simulink model "tutorial_vms"  (R2023a)
settings: Solver=FixedStepAuto  StartTime=0.0  StopTime=50  FixedStep=framePeriod_s  RelTol=1e-3
undefined symbols (not defined in the file): Aircraft, framePeriod_s
settings Model: Creator=brian  LastModifiedBy=tuan
settings SolverCC: AlgebraicLoopSolver=TrustRegion
settings OptimizationCC: DefaultParameterBehavior=Inlined  GainParamInheritBuiltInType=on  UseFloatMulNetSlope=on  DefaultUnderspecifiedDataType=single  EnhancedBackFolding=on  BooleansAsBitfields=on  PassReuseOutputArgsAs=Individual arguments  StateBitsets=on  DataBitsets=on  ActiveStateOutputEnumStorageType=uint16  ZeroExternalMemoryAtStartup=off  ZeroInternalMemoryAtStartup=off  EfficientFloat2IntCast=on  LifeSpan=inf  DifferentSizesBufferReuse=on  OptimizationPriority=RAM  OptimizationCustomize=off  EfficientTunableParamExpr=on
settings DebuggingCC: ParameterPrecisionLossMsg=none  ParameterTunabilityLossMsg=error  UnconnectedInputMsg=warning  UnconnectedOutputMsg=warning  UnconnectedLineMsg=warning  BusObjectLabelMismatch=error  RootOutportRequireBusObject=error  NonBusSignalsTreatedAsBus=error  SFInvalidInputDataAccessInChartInitDiag=error  SFTransitionOutsideNaturalParentDiag=error  SFUnreachableExecutionPathDiag=error  SFUndirectedBroadcastEventsDiag=error
settings HardwareCC: ProdBitPerPointer=32  ProdBitPerSizeT=32  ProdBitPerPtrDiffT=32  ProdLargestAtomicInteger=Long  ProdLargestAtomicFloat=Double  ProdWordSize=32  ProdHWDeviceType=NXP->Cortex-M4  TargetLargestAtomicInteger=Long  TargetLargestAtomicFloat=Double  TargetLongLongMode=on  TargetIntDivRoundTo=Zero  TargetEndianess=LittleEndian  TargetHWDeviceType=NXP->Cortex-M4  ProdEqTarget=off
settings ModelReferenceCC: EnableRefExpFcnMdlSchedulingChecks=on  ModelReferenceNumInstancesAllowed=Single
settings SFSimCC: SimParseCustomCode=off  SimGenImportedTypeDefs=on  MATLABDynamicMemAlloc=off  SimTargetLang=C++
settings SFSimCC: SimUserIncludeDirs=|
  | ../../flight_code/include
  | ../../../ua_spaaro_extra/imu/include
  | ../../../ua_spaaro_extra/gnss/include
  | ../../../ua_spaaro_extra/pres/include
  | ../../../ua_spaaro_extra/sbus/include
  | ../../../ua_spaaro_extra/global_defs/include
settings SFSimCC: SimUserDefines=|
  | SIL
  | __FMU_R_MINI_V1__
settings RTWCC: Description=Embedded Coder  SystemTargetFile=ert.tlc  GenCodeOnly=on  TemplateMakefile=ert_default_tmf  GenerateReport=on  RTWVerbose=off  RTWUseSimCustomCode=on  Toolchain=GNU gcc/g++ | gmake (64-bit Linux)  BuildConfiguration=Specify  IncludeHyperlinkInReport=on  LaunchReport=on  TargetLang=C++  GenerateTraceInfo=on  GenerateTraceReport=on  GenerateTraceReportSl=on  GenerateTraceReportSf=on  GenerateTraceReportEml=on  GenerateCodeReplacementReport=on  DLArmComputeVersion=19.05
settings RTWCC: CustomInclude=|
  | ../../flight_code/include
  | ../../../ua_spaaro_extra/imu/include
  | ../../../ua_spaaro_extra/gnss/include
  | ../../../ua_spaaro_extra/pres/include
  | ../../../ua_spaaro_extra/sbus/include
  | ../../../ua_spaaro_extra/global_defs/include
settings RTWCC: CustomDefine=|
  | SIL
  | __FMU_R_MINI_V1__
settings CodeAppCC: ForceParamTrailComments=on  IgnoreCustomStorageClasses=off  OperatorAnnotations=on  SimulinkDataObjDesc=on  SFDataObjDesc=on  MATLABFcnDesc=on  CustomSymbolStrGlobalVar=rt$N$M  CustomSymbolStrType=$N$M  CustomSymbolStrFcn=$N$M$F  CustomSymbolStrMacro=$N$M  InsertBlockDesc=on  StateflowObjectComments=on  MATLABSourceComments=on  EnableCustomComments=on  InternalIdentifier=Classic  InlinedPrmAccess=Macros  ReqsInCode=on
settings ERTTargetCC: TargetLangStandard=C++03 (ISO)  GenerateFullHeader=off  IncludeMdlTerminateFcn=off  CombineSignalStateStructs=on  SuppressErrorStatus=on  SupportAbsoluteTime=off  CodeInterfacePackaging=C++ class  SupportNonFinite=off  SupportComplex=off  ParenthesesLevel=Standards  CastingMode=Standards  ERTHeaderFileRootName=autocode$E  ERTSourceFileRootName=autocode$E  InlinedParameterPlacement=NonHierarchical  RootIOFormat=Structure reference  ERTCustomFileTemplate=example_file_process.tlc  ERTFilePackagingFormat=Compact  PreserveExpressionOrder=on  PreserveIfCondition=on  ConvertIfToSwitch=off  EnableSignedLeftShifts=off  EnableSignedRightShifts=off  IndentSize=4

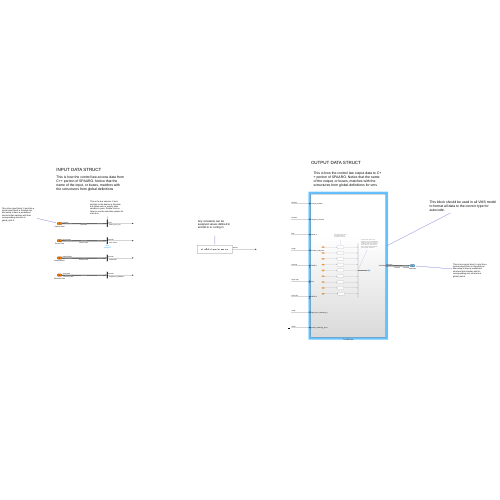
[thumbnail: Simulink's stored preview of the top-level diagram]
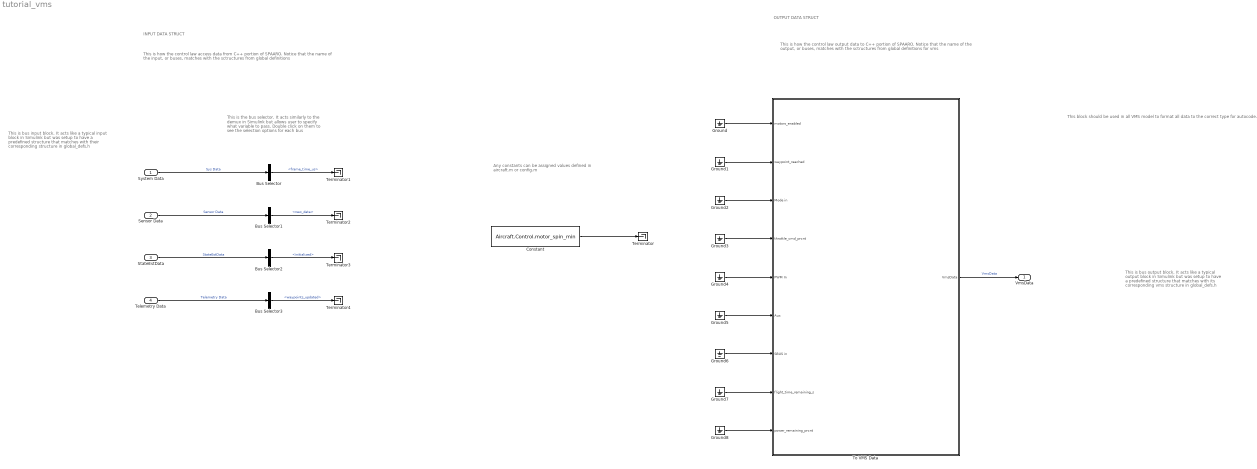
== system tutorial_vms ==
  note: This is bus input block. It acts like a typical input block in Simulink but was setup to have a predefined structure that matches with their corresponding structure in global_defs.h
  note: This is how the control law access data from C++ portion of SPAARO. Notice that the name of the input, or buses, matches with the sctructures from global definitions
  note: INPUT DATA STRUCT
  note: This is the bus selector. It acts similarly to the demux in Simulink but allows user to specify what variable to pass. Double click on them to see the selection options for each bus
  note: Any constants can be assigned values defined in aircraft.m or config.m
  note: OUTPUT DATA STRUCT
  note: This block should be used in all VMS model to format all data to the correct type for autocode.
  note: This is how the control law output data to C++ portion of SPAARO. Notice that the name of the output, or buses, matches with the sctructures from global definitions for vms
  note: This is bus output block. It acts like a typical output block in Simulink but was setup to have a predefined structure that matches with its corresponding vms structure in global_defs.h
  System Data : Inport  OutDataTypeStr=Bus: SysData  SampleTime=framePeriod_s  BusOutputAsStruct=on
  Sensor Data : Inport  Port=2  OutDataTypeStr=Bus: SensorData  SampleTime=framePeriod_s  BusOutputAsStruct=on
  StateEstData : Inport  Port=3  OutDataTypeStr=Bus: StateEstData  SampleTime=framePeriod_s  BusOutputAsStruct=on
  Telemetry Data : Inport  Port=4  OutDataTypeStr=Bus: TelemData  SampleTime=framePeriod_s  BusOutputAsStruct=on
  Bus Selector : BusSelector  OutputSignals=frame_time_us
  Bus Selector1 : BusSelector  OutputSignals=inceptor.new_data
  Bus Selector2 : BusSelector  OutputSignals=bfs_ins.initialized
  Bus Selector3 : BusSelector  OutputSignals=waypoints_updated
  Constant : Constant  Value=Aircraft.Control.motor_spin_min
  Ground{,1..8} (9 alike) : Ground
  Terminator{,1..4} (5 alike) : Terminator
  To VMS Data : Subsystem
  VmsData : Outport  OutDataTypeStr=Bus: VmsData  SampleTime=framePeriod_s  BusOutputAsStruct=on
  wires:
  To VMS Data/1(VmsData) -> VmsData/1  "VmsData"
  System Data/1 -> Bus Selector/1  "Sys Data"
  Sensor Data/1 -> Bus Selector1/1  "Sensor Data"
  StateEstData/1 -> Bus Selector2/1  "StateEstData"
  Telemetry Data/1 -> Bus Selector3/1  "Telemetry Data"
  Ground/1 -> To VMS Data/1(motors_enabled)
  Constant/1 -> Terminator/1
  Bus Selector/1 -> Terminator1/1  "<frame_time_us>"
  Bus Selector3/1 -> Terminator4/1  "<waypoints_updated>"
  Bus Selector2/1 -> Terminator3/1  "<initialized>"
  Bus Selector1/1 -> Terminator2/1  "<new_data>"
  Ground1/1 -> To VMS Data/2(waypoint_reached)
  Ground2/1 -> To VMS Data/3(Mode in)
  Ground3/1 -> To VMS Data/4(throttle_cmd_prcnt)
  Ground4/1 -> To VMS Data/5(PWM In)
  Ground5/1 -> To VMS Data/6(Aux)
  Ground6/1 -> To VMS Data/7(SBUS in)
  Ground7/1 -> To VMS Data/8(flight_time_remaining_s)
  Ground8/1 -> To VMS Data/9(power_remaining_prcnt)

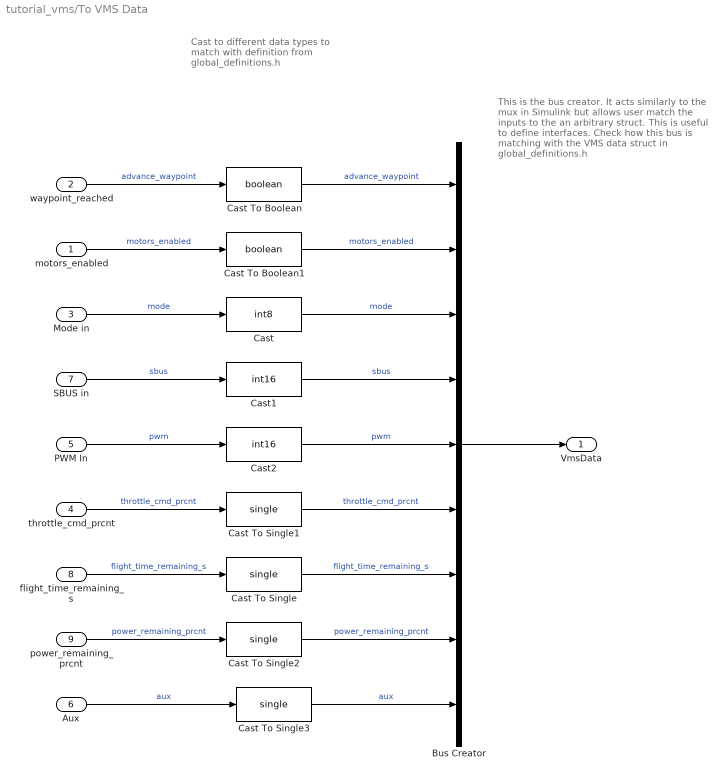
== system tutorial_vms/To VMS Data ==
  note: Cast to different data types to match with definition from global_definitions.h
  note: This is the bus creator. It acts similarly to the mux in Simulink but allows user match the inputs to the an arbitrary struct. This is useful to define interfaces. Check how this bus is matching with the VMS data struct in global_definitions.h
  motors_enabled : Inport
  waypoint_reached : Inport  Port=2
  Mode in : Inport  Port=3
  throttle_cmd_prcnt : Inport  Port=4
  PWM In : Inport  Port=5
  Aux : Inport  Port=6
  SBUS in : Inport  Port=7
  flight_time_remaining_s : Inport  Port=8
  power_remaining_prcnt : Inport  Port=9
  Bus Creator : BusCreator  Inputs=9  OutDataTypeStr=Bus: VmsData  NonVirtualBus=on
      settings: InheritFromInputs=off
  Cast : DataTypeConversion  OutDataTypeStr=int8  SaturateOnIntegerOverflow=off  RndMeth=Floor
  Cast To Boolean : DataTypeConversion  OutDataTypeStr=boolean  SaturateOnIntegerOverflow=off  RndMeth=Floor
  Cast To Boolean1 : DataTypeConversion  OutDataTypeStr=boolean  SaturateOnIntegerOverflow=off  RndMeth=Floor
  Cast To Single{,1..3} (4 alike) : DataTypeConversion  OutDataTypeStr=single  SaturateOnIntegerOverflow=off  RndMeth=Floor
  Cast1 : DataTypeConversion  OutDataTypeStr=int16  SaturateOnIntegerOverflow=off  RndMeth=Floor
  Cast2 : DataTypeConversion  OutDataTypeStr=int16  SaturateOnIntegerOverflow=off  RndMeth=Floor
  VmsData : Outport
  wires:
  Bus Creator/1 -> VmsData/1
  waypoint_reached/1 -> Cast To Boolean/1  "advance_waypoint"
  motors_enabled/1 -> Cast To Boolean1/1  "motors_enabled"
  Mode in/1 -> Cast/1  "mode"
  SBUS in/1 -> Cast1/1  "sbus"
  PWM In/1 -> Cast2/1  "pwm"
  throttle_cmd_prcnt/1 -> Cast To Single1/1  "throttle_cmd_prcnt"
  Aux/1 -> Cast To Single3/1  "aux"
  Cast To Single2/1 -> Bus Creator/8  "power_remaining_prcnt"
  Cast To Single/1 -> Bus Creator/7  "flight_time_remaining_s"
  flight_time_remaining_s/1 -> Cast To Single/1  "flight_time_remaining_s"
  Cast To Boolean/1 -> Bus Creator/1  "advance_waypoint"
  Cast To Boolean1/1 -> Bus Creator/2  "motors_enabled"
  Cast/1 -> Bus Creator/3  "mode"
  Cast1/1 -> Bus Creator/4  "sbus"
  Cast2/1 -> Bus Creator/5  "pwm"
  Cast To Single1/1 -> Bus Creator/6  "throttle_cmd_prcnt"
  power_remaining_prcnt/1 -> Cast To Single2/1  "power_remaining_prcnt"
  Cast To Single3/1 -> Bus Creator/9  "aux"
